simulink model "PBVS"  (R2020b)
settings: Solver=VariableStepAuto  StartTime=0.0  StopTime=7  RelTol=1e-3
values from neighbouring files (symbols this model uses):
  beta = 0.01    [init_PBVS.m]
  dT = 1/frequency    (= 0.005)    [init.m]    (also in init_PBVS.m = 0.002)
  DT = 1/20    (= 0.05)    [init_PBVS.m]
  f = 0.5    [init.m]    (also in init_PBVS.m = 0.1; robotIK.m = zeros(3,1))
  init_pose = [C ; ang']    [init.m]    (also in init_PBVS.m = [position(1:3); orientation'])
  Kd = 0.1*eye(6)    [init_PBVS.m]
  Kp = 1*eye(6)    [init.m]    (also in init_PBVS.m = diag([4 4 4 1.5 1.5 1.5]))
  N = 10    [init_PBVS.m]    (also in robotIK.m = size(jointLim, 1); workspace.m = 50)
  O = [0; 0; 0]    [init.m]    (also in init_PBVS.m)
  p = [0.25; 0; 0.25]    [init_PBVS.m]
  P0 = eye(6)*0.5    [init_PBVS.m]
  plane_x = 0.1    [init_PBVS.m]
  plane_y = 0.08    [init_PBVS.m]
  q = [0. 0. 0. -pi/2 0. pi/2 0. 0 0.]    [init_PBVS.m]    (also in robotIK.m = real(qToCheck))
  Q = zeros(6)    [init_PBVS.m]
  ref = [-0.2; 0; 0; pi/2; 0 ; pi/2]    [init.m]    (also in init_PBVS.m = [0; 0; 0.15; 0;  0; -pi])
libraries: simulink x2, robotmaniplib x2, cstblocks x1
settings Model: Creator=Acer  LastModifiedBy=antonio

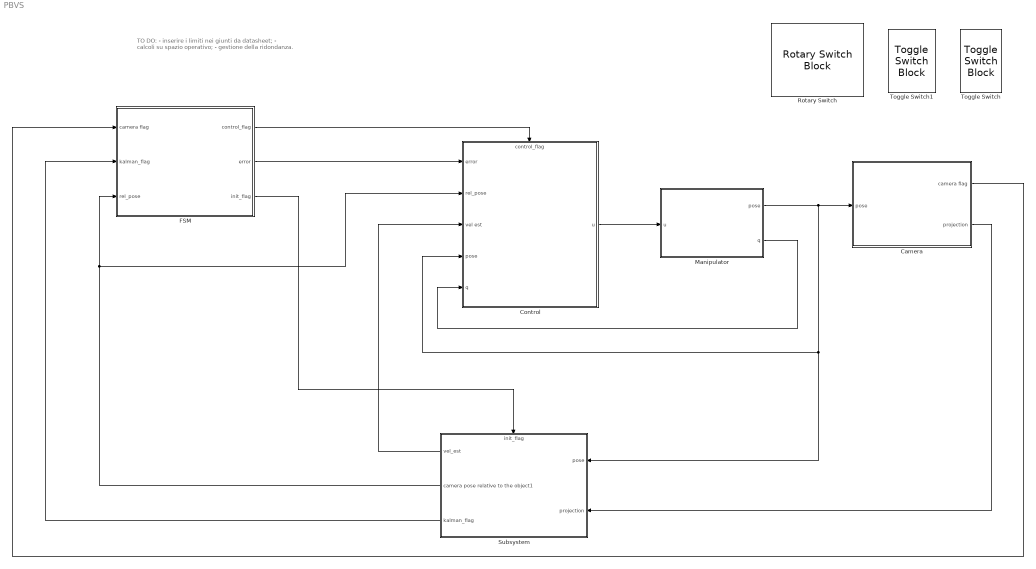
== system PBVS ==
  note: TO DO:
      | - inserire i limiti nei giunti da datasheet;
      | - calcoli su spazio operativo;
      | - gestione della ridondanza.
  Camera : Subsystem
  Control : Subsystem
      settings: PortSchema="{\"entries\":[{\"content\":{\"sides\":[{\"content\":{\"connectorIds\":[\"In1\",\"In2\",\"In3\",\"In4\",\"In5\"]},\"type\":\"ConnectorPlacement.EquallySpacedRectSide\",\"uuid\":\"af17fae2-36f6-4efd-b4ba-fb8d1f73429e\"},{\"content\":{\"connectorIds\":[\"Out1\"],\"side\":\"RIGHT\"},\"type\":\"ConnectorPlacement.EquallySpacedRectSide\",\"uuid\":\"2b8fdab6-bdef-4319-b746-176742d42689\"},{\"content\":{\"connectorIds\":[\"In6\"],\"side\":\"TOP\"},\"type\":\"ConnectorPlacement.EquallySpacedRectSide\",\"uuid\":\"e47b4a6a-66e6-45a0-98f9-e5ee84c20568\"},{\"content\":{\"connectorIds\":[],\"side\":\"HIDDEN\"},\"type\":\"ConnectorPlacement.EquallySpacedRectSide\",\"uuid\":\"9d3dc715-f15e-4844-9864-7097570c16fc\"}]},\"type\":\"ConnectorPlacement.EquallySpacedConnector\",\"uuid\":\"752007b5-316d-48d1-9942-1c7a203faf23\"}],\"packageUris\":[\"http://schema.mathworks.com/mf0/Connector/R2020b\"],\"version\":\"1.0\"}"
  FSM : Subsystem
  Manipulator : Subsystem
  Rotary Switch : RotarySwitchBlock  LabelPosition=Bottom
      settings: Values={{'Off', 'Low', 'Medium', 'High'}, [0 -0.03 -0.06 -0.1]}
  Subsystem : Subsystem
      settings: PortSchema="{\"entries\":[{\"content\":{\"sides\":[{\"content\":{\"connectorIds\":[\"In1\",\"In2\"]},\"type\":\"ConnectorPlacement.EquallySpacedRectSide\",\"uuid\":\"a08c32dc-abe6-4f2b-ae77-c4d2f876d1ca\"},{\"content\":{\"connectorIds\":[\"Out1\",\"Out2\",\"Out3\"],\"side\":\"RIGHT\"},\"type\":\"ConnectorPlacement.EquallySpacedRectSide\",\"uuid\":\"a9594212-1ad7-4004-b7e9-4ae8430051bc\"},{\"content\":{\"connectorIds\":[\"In3\"],\"side\":\"TOP\"},\"type\":\"ConnectorPlacement.EquallySpacedRectSide\",\"uuid\":\"c64d48d0-945a-48a3-9b1a-7425a2bac4f1\"},{\"content\":{\"connectorIds\":[],\"side\":\"HIDDEN\"},\"type\":\"ConnectorPlacement.EquallySpacedRectSide\",\"uuid\":\"141999d7-d8a1-4566-a0df-60055f832239\"}]},\"type\":\"ConnectorPlacement.EquallySpacedConnector\",\"uuid\":\"574f16a2-9616-413e-b861-7d1dd0d71272\"}],\"packageUris\":[\"http://schema.mathworks.com/mf0/Connector/R2020b\"],\"version\":\"1.0\"}"
  Toggle Switch : ToggleSwitchBlock  LabelPosition=Bottom
      settings: Values={{'Off', 'On'}, [0 1]}
  Toggle Switch1 : ToggleSwitchBlock  LabelPosition=Bottom
      settings: Values={{'Off', 'On'}, [0 1]}
  wires:
  Camera/2(projection) -> Subsystem/2(projection)
  Control/1(u) -> Manipulator/1(u)
  Manipulator/1(pose) -> Subsystem/1(pose), Control/4(pose), Camera/1(pose)
  Manipulator/2(q) -> Control/5(q)
  Subsystem/2(camera pose relative to the object1) -> FSM/3(rel_pose), Control/2(rel_pose)
  Subsystem/1(vel_est) -> Control/3(vel est)
  FSM/2(error) -> Control/1(error)
  Subsystem/3(kalman_flag) -> FSM/2(kalman_flag)
  FSM/1(control_flag) -> Control/6(control_flag)
  FSM/3(init_flag) -> Subsystem/3(init_flag)
  Camera/1(camera flag) -> FSM/1(camera flag)

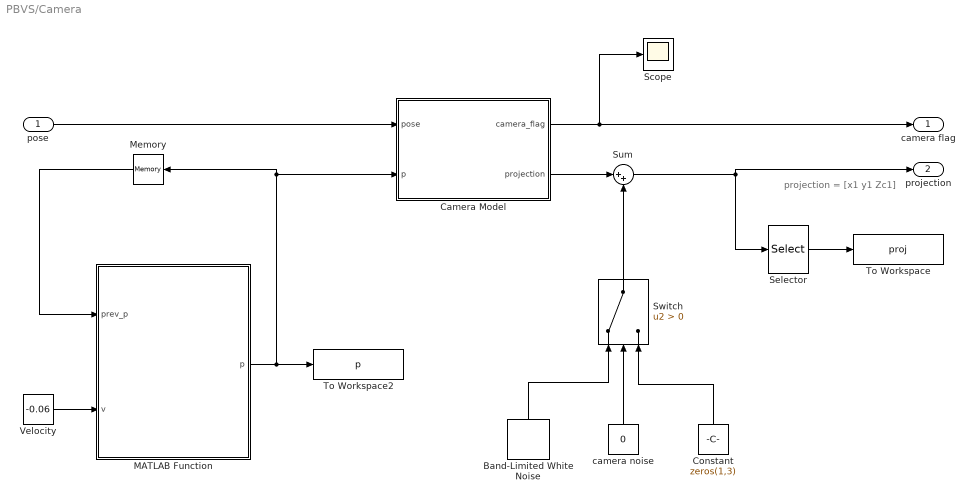
== system PBVS/Camera ==
  note: projection = [x1 y1 Zc1]
  pose : Inport
  Band-Limited White Noise : simulink/Sources/Band-Limited White Noise  Cov=[0.000001 0.000001 0.000001]  Ts=0.01  seed=[23341 10 14]
  Camera Model : MATLAB Function  TreatAsAtomicUnit=on
  Constant : Constant  Value=zeros(1,3)
  MATLAB Function : MATLAB Function  TreatAsAtomicUnit=on  SystemSampleTime=dT
  Memory : Memory  InitialCondition=[p]
  Scope : Scope
  Selector : Selector  InputPortWidth=3  IndexOptions=Index vector (dialog)  Indices=[1 2]  OutputSizes=1
  Sum : Sum  Inputs=|++
  Switch : Switch  Criteria=u2 > Threshold
  To Workspace : ToWorkspace  VariableName=proj  SampleTime=0.1
  To Workspace2 : ToWorkspace  VariableName=p  SampleTime=0.1
  Velocity : Constant  Value=-0.06  SampleTime=dT
  camera noise : Constant  Value=0
  camera flag : Outport
  projection : Outport  Port=2
  wires:
  pose/1 -> Camera Model/1(pose)
  Selector/1 -> To Workspace/1
  Camera Model/2(projection) -> Sum/1
  Sum/1 -> projection/1, Selector/1
  Switch/1 -> Sum/2
  camera noise/1 -> Switch/2
  Band-Limited White Noise/1 -> Switch/1
  Constant/1 -> Switch/3
  MATLAB Function/1(p) -> To Workspace2/1, Memory/1, Camera Model/2(p)
  Memory/1 -> MATLAB Function/1(prev_p)
  Velocity/1 -> MATLAB Function/2(v)
  Camera Model/1(camera_flag) -> Scope/1, camera flag/1

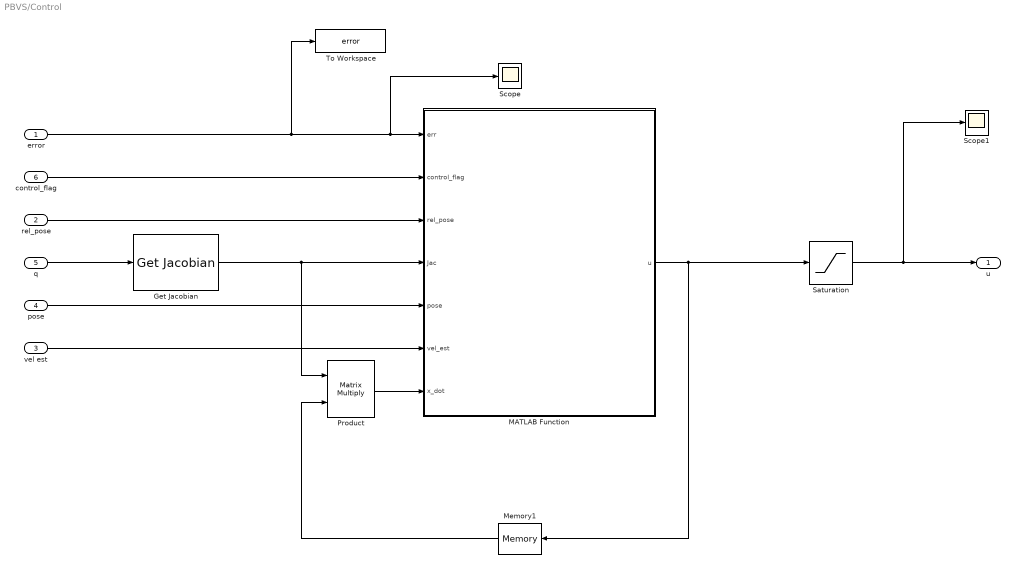
== system PBVS/Control ==
  error : Inport
  rel_pose : Inport  Port=2
  vel est : Inport  Port=3
  pose : Inport  Port=4
  q : Inport  Port=5
  control_flag : Inport  Port=6
  Get Jacobian : robotmaniplib/Get Jacobian  RigidBodyTree=robot  EndEffector=panda_hand  SimulateUsing=Interpreted execution
      settings: SourceProductBaseCode=RO
  MATLAB Function : MATLAB Function  TreatAsAtomicUnit=on  SystemSampleTime=dT
  Memory1 : Memory  InitialCondition=zeros(9,1)
  Product : Product  Multiplication=Matrix(*)
  Saturation : Saturate  UpperLimit=2.5  LowerLimit=-2.5
  Scope : Scope
  Scope1 : Scope
  To Workspace : ToWorkspace  VariableName=error  SampleTime=0.1
  u : Outport
  wires:
  error/1 -> To Workspace/1, Scope/1, MATLAB Function/1(err)
  rel_pose/1 -> MATLAB Function/3(rel_pose)
  MATLAB Function/1(u) -> Memory1/1, Saturation/1
  q/1 -> Get Jacobian/1
  Get Jacobian/1 -> Product/1, MATLAB Function/4(Jac)
  Saturation/1 -> Scope1/1, u/1
  pose/1 -> MATLAB Function/5(pose)
  Product/1 -> MATLAB Function/7(x_dot)
  Memory1/1 -> Product/2
  vel est/1 -> MATLAB Function/6(vel_est)
  control_flag/1 -> MATLAB Function/2(control_flag)

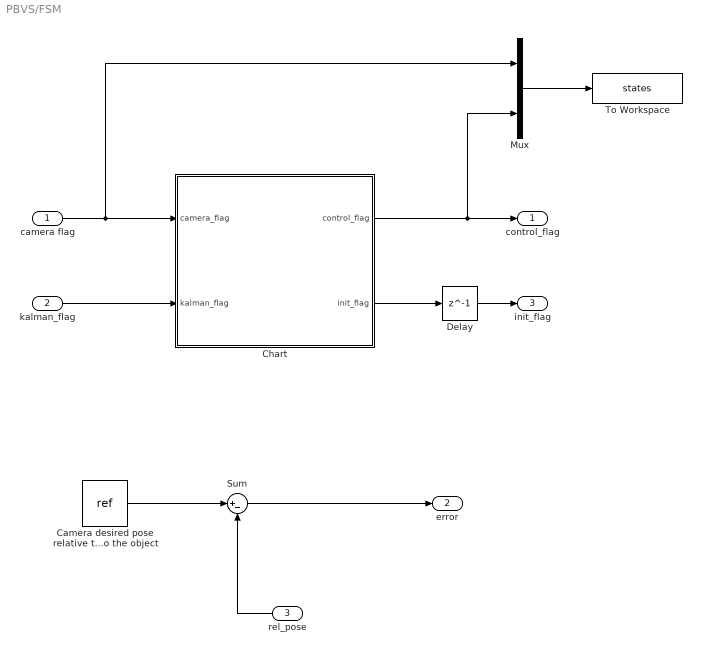
== system PBVS/FSM ==
  camera flag : Inport
  kalman_flag : Inport  Port=2
  rel_pose : Inport  Port=3
  Camera desired pose relative to the object : Constant  Value=ref  SampleTime=-1
  Chart : Stateflow chart  TreatAsAtomicUnit=on
  Delay : Delay  DelayLength=1
  Mux : Mux  Inputs=2
  Sum : Sum  Inputs=|+-
  To Workspace : ToWorkspace  VariableName=states  SampleTime=0.1
  control_flag : Outport
  error : Outport  Port=2
  init_flag : Outport  Port=3
  wires:
  Sum/1 -> error/1
  Camera desired pose relative to the object/1 -> Sum/1
  rel_pose/1 -> Sum/2
  kalman_flag/1 -> Chart/2(kalman_flag)
  Chart/1(control_flag) -> Mux/2, control_flag/1
  camera flag/1 -> Chart/1(camera_flag), Mux/1
  Chart/2(init_flag) -> Delay/1
  Delay/1 -> init_flag/1
  Mux/1 -> To Workspace/1

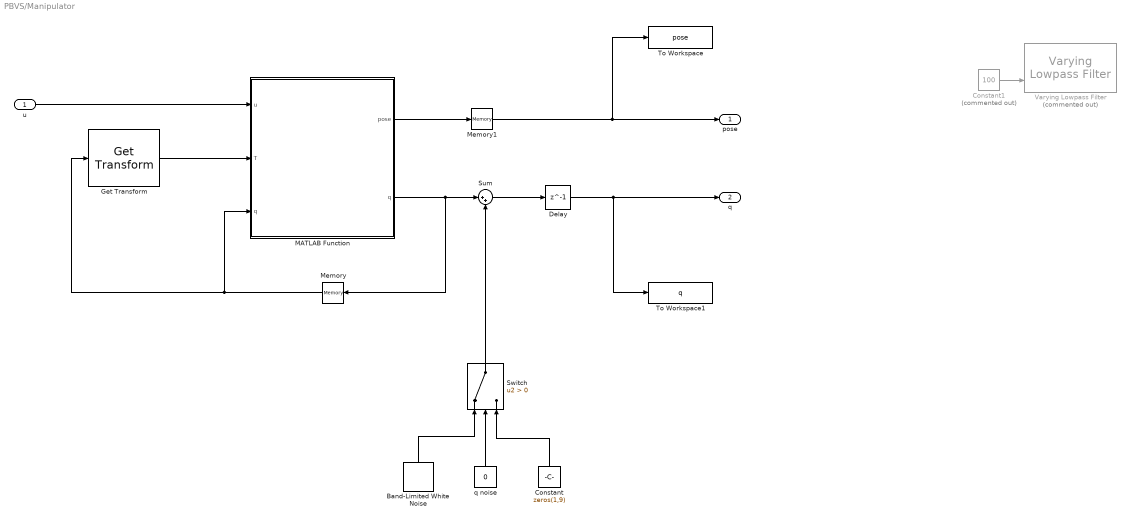
== system PBVS/Manipulator ==
  u : Inport
  Band-Limited White Noise : simulink/Sources/Band-Limited White Noise  Cov=[0.000001 0.000001 0.000001 0.000001 0.000001 0.000001 0.000001 0.0 0.0]  Ts=0.01  seed=[3341 17 144 12 1 94 2456 78 91]
  Constant : Constant  Value=zeros(1,9)
  Constant1 : Constant  Commented=on  Value=100
  Delay : Delay  DelayLength=1
  Get Transform : robotmaniplib/Get Transform  RigidBodyTree=robot  SourceBody=panda_link0  TargetBody=panda_hand  SimulateUsing=Interpreted execution
  MATLAB Function : MATLAB Function  TreatAsAtomicUnit=on  SystemSampleTime=dT
  Memory : Memory  InitialCondition=q
  Memory1 : Memory  InitialCondition=init_pose
  Sum : Sum  Inputs=|++
  Switch : Switch  Criteria=u2 > Threshold
  To Workspace : ToWorkspace  VariableName=pose  SampleTime=0.1
  To Workspace1 : ToWorkspace  VariableName=q  SampleTime=0.1
  Varying Lowpass Filter : cstblocks/Linear Parameter Varying/Varying Lowpass Filter  Commented=on  N=1
  q noise : Constant  Value=0
  pose : Outport
  q : Outport  Port=2
  wires:
  Memory/1 -> MATLAB Function/3("q "), Get Transform/1
  Get Transform/1 -> MATLAB Function/2(T)
  MATLAB Function/1(pose) -> Memory1/1
  Memory1/1 -> pose/1, To Workspace/1
  u/1 -> MATLAB Function/1(u)
  Constant/1 -> Switch/3
  Band-Limited White Noise/1 -> Switch/1
  Switch/1 -> Sum/2
  q noise/1 -> Switch/2
  MATLAB Function/2(q) -> Memory/1, Sum/1
  Sum/1 -> Delay/1
  Delay/1 -> q/1, To Workspace1/1
  Constant1/1 -> Varying Lowpass Filter/2

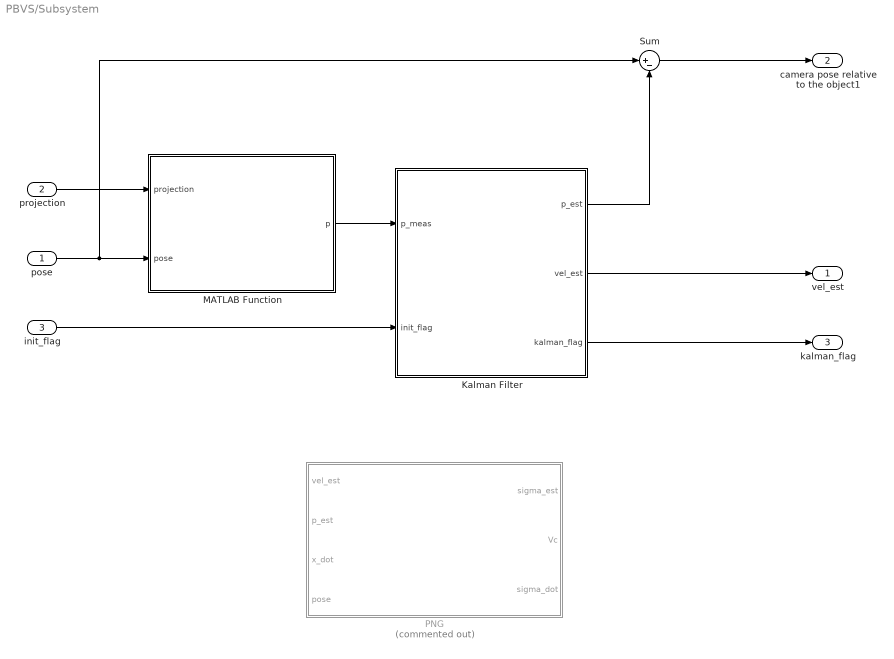
== system PBVS/Subsystem ==
  pose : Inport
  projection : Inport  Port=2
  init_flag : Inport  Port=3
  Kalman Filter : Subsystem
  MATLAB Function : MATLAB Function  TreatAsAtomicUnit=on
  PNG : Subsystem  Commented=on
  Sum : Sum  Inputs=|+-
  vel_est : Outport
  camera pose relative to the object1 : Outport  Port=2
  kalman_flag : Outport  Port=3
  wires:
  projection/1 -> MATLAB Function/1(projection)
  MATLAB Function/1(p) -> Kalman Filter/1(p_meas)
  Kalman Filter/2(vel_est) -> vel_est/1
  pose/1 -> Sum/1, MATLAB Function/2(pose)
  Sum/1 -> camera pose relative to the object1/1
  Kalman Filter/1(p_est) -> Sum/2
  Kalman Filter/3(kalman_flag) -> kalman_flag/1
  init_flag/1 -> Kalman Filter/2(init_flag)

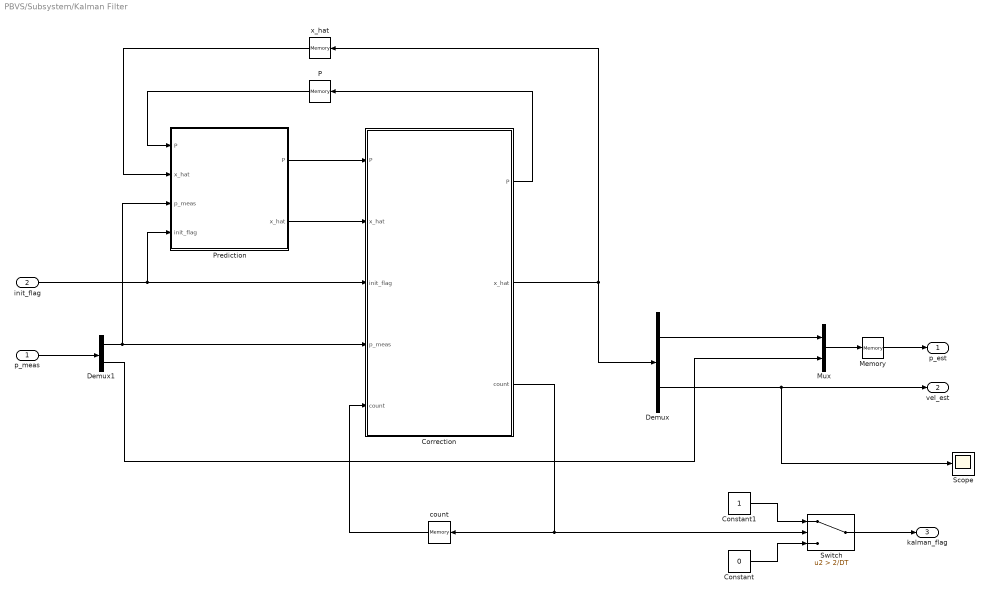
== system PBVS/Subsystem/Kalman Filter ==
  p_meas : Inport
  init_flag : Inport  Port=2
  Constant : Constant  Value=0
  Constant1 : Constant
  Correction : MATLAB Function  TreatAsAtomicUnit=on  SystemSampleTime=DT
  Demux : Demux  Outputs=2
  Demux1 : Demux  Outputs=2
  Memory : Memory  InitialCondition=zeros(6,1)
  Mux : Mux  Inputs=2
  P : Memory  InitialCondition=P0
  Prediction : MATLAB Function  TreatAsAtomicUnit=on  SystemSampleTime=DT
  Scope : Scope
  Switch : Switch  Criteria=u2 > Threshold  Threshold=2/DT
  count : Memory
  x_hat : Memory  InitialCondition=[p; zeros(3,1)]
  p_est : Outport
  vel_est : Outport  Port=2
  kalman_flag : Outport  Port=3
  wires:
  Demux/2 -> Scope/1, vel_est/1
  x_hat/1 -> Prediction/2("x_hat ")
  P/1 -> Prediction/1("P ")
  Correction/2(x_hat) -> x_hat/1, Demux/1
  Correction/1(P) -> P/1
  Prediction/1(P) -> Correction/1("P ")
  Prediction/2(x_hat) -> Correction/2("x_hat ")
  p_meas/1 -> Demux1/1
  Mux/1 -> Memory/1
  Demux/1 -> Mux/1
  Demux1/1 -> Prediction/3(p_meas), Correction/4(p_meas)
  Demux1/2 -> Mux/2
  Memory/1 -> p_est/1
  Correction/3(count) -> count/1, Switch/2
  count/1 -> Correction/5("count ")
  Constant/1 -> Switch/3
  Constant1/1 -> Switch/1
  Switch/1 -> kalman_flag/1
  init_flag/1 -> Prediction/4(init_flag), Correction/3(init_flag)

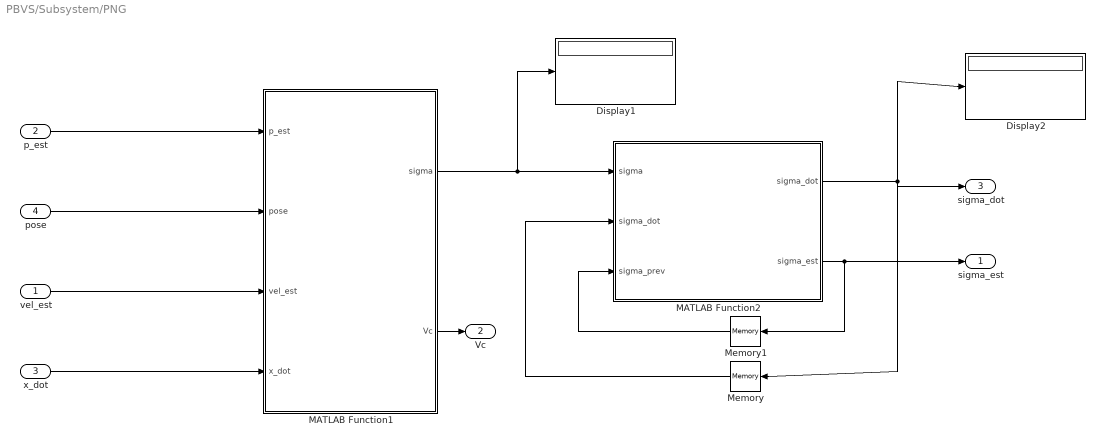
== system PBVS/Subsystem/PNG ==
  vel_est : Inport
  p_est : Inport  Port=2
  x_dot : Inport  Port=3
  pose : Inport  Port=4
  Display1 : Display
  Display2 : Display
  MATLAB Function1 : MATLAB Function  TreatAsAtomicUnit=on
  MATLAB Function2 : MATLAB Function  TreatAsAtomicUnit=on  SystemSampleTime=DT
  Memory : Memory  InitialCondition=zeros(3,1)
  Memory1 : Memory  InitialCondition=zeros(3,1)
  sigma_est : Outport
  Vc : Outport  Port=2
  sigma_dot : Outport  Port=3
  wires:
  MATLAB Function1/2(Vc) -> Vc/1
  MATLAB Function2/2(sigma_est) -> sigma_est/1, Memory1/1
  MATLAB Function1/1(sigma) -> Display1/1, MATLAB Function2/1(sigma)
  pose/1 -> MATLAB Function1/2(pose)
  Memory/1 -> MATLAB Function2/2("sigma_dot ")
  MATLAB Function2/1(sigma_dot) -> sigma_dot/1, Display2/1, Memory/1
  Memory1/1 -> MATLAB Function2/3(sigma_prev)
  x_dot/1 -> MATLAB Function1/4(x_dot)
  p_est/1 -> MATLAB Function1/1(p_est)
  vel_est/1 -> MATLAB Function1/3(vel_est)

== stateflow chart PBVS/FSM/Chart ==
  state Stop
    entry:
    control_flag = 0;
    init_flag = 0;
  state ComputeSpeed
    entry:
    control_flag = 0;
    init_flag = 1;
  state GraspTheObject
    entry:
    control_flag = 1;
  (default) -> Stop
  ComputeSpeed -> Stop [order 2] : [camera_flag == 0]
  Stop -> ComputeSpeed : [camera_flag == 1]
  ComputeSpeed -> GraspTheObject [order 1] : [kalman_flag == 1]
  data: camera_flag input; kalman_flag input; control_flag output; init_flag output

== matlab function PBVS/Subsystem/PNG/MATLAB Function2 ==
  data: sigma input; sigma_dot output; sigma_dot input; sigma_prev input; sigma_est output; DT parameter; beta parameter
function [sigma_dot, sigma_est] = fading_filter(sigma, sigma_dot, sigma_prev, DT, beta)

G = 1 - beta^2;
H = (1 - beta)^2;
sigma_est = zeros(3,1);

sigma_est = sigma_prev + sigma_dot * DT + G * (sigma - (sigma_prev + sigma_dot*DT));
sigma_dot = sigma_dot + H/DT * (sigma - (sigma_prev + sigma_dot * DT))

== matlab function PBVS/Subsystem/Kalman Filter/Correction ==
  data: P input; P output; x_hat input; init_flag input; x_hat output; p_meas input; count input; R parameter; count output
function [P, x_hat, count] = correction(P, x_hat, init_flag,p_meas, count, R)

if init_flag == 1
C = [eye(3) zeros(3); zeros(3) zeros(3)];
z = [p_meas; zeros(3,1)];

K = P * C' * (C * P * C' + R)^-1;
x_hat = x_hat + K * (z - C * x_hat);
P = (eye(6) - K * C) * P;

count = count + 1;
end

== matlab function PBVS/Subsystem/Kalman Filter/Prediction ==
  data: P input; P output; x_hat input; p_meas input; x_hat output; Q parameter; DT parameter; init_flag input
function [P, x_hat] = prediction(P, x_hat, p_meas, Q, DT, init_flag)

if init_flag == 1
A = [eye(3) DT*eye(3); zeros(3) eye(3)];

x_hat = A * x_hat;
P = A * P * A' + Q;
end

== matlab function PBVS/Control/MATLAB Function ==
  data: err input; control_flag input; rel_pose input; Jac input; Kp parameter; u output; ref parameter; pose input; vel_est input; x_dot input; Kd parameter; dT parameter; N parameter
function u = fcn(err, control_flag, rel_pose, Jac, Kp, ref, pose, vel_est, x_dot, Kd, dT, N)

% rel_pose : relative pose between camera and object
% ref : desired relative pose between camera and object
% err : error between desired and actual pose of the camera relative to the object
u = zeros(9, 1);

if (control_flag == 1)

    ang = zeros(3, 1);
    J = zeros(6, 9);
    ang(1) = rel_pose(4) - ref(4);  % camera's orientation 
    ang(2) = rel_pose(5) - ref(5);
    ang(3) = rel_pose(6) - ref(6);

    %% Trasformation
    Rx = [1   0       0   ;
          0 cos(ang(1)) -sin(ang(1));
          0 sin(ang(1)) cos(ang(1))];

    Ry = [cos(ang(2)) 0 sin(ang(2)) ;
           0     1   0    ;
         -sin(ang(2)) 0 cos(ang(2))];

    Rz = [cos(ang(3)) -sin(ang(3)) 0;
          sin(ang(3))  cos(ang(3)) 0;
           0      0     1];

    Rd = Rz * Ry * Rx; % rotation matrix 

    J2 = [1     sin(ang(1))*tan(ang(2))    cos(ang(1))*tan(ang(2));
          0           cos(ang(1))                  -sin(ang(1));
          0     sin(ang(1))/cos(ang(2))    cos(ang(1))/cos(ang(2)) ];

    Ta = [0     -sin(pose(1))       cos(pose(1))*sin(pose(2));
          0      cos(pose(1))       sin(pose(1))*sin(pose(2));
          1          0                        cos(pose(2))];

    if (det(Ta)==0)
        Ta = eye(3);
    end

    %% Jacobian
    %J = eye(6);  % Jacobian J(q)
    J(1:3, :) = Jac(4:6, :);
    J(4:6, :) = Jac(1:3, :);
    %
    Ja = [eye(3) zeros(3); zeros(3) Rd'*Ta^-1] * J;
    %null_Ja = null(Ja);

    %% PBVS control Law
    % n = zeros(3,1);    % end effector acceleration in xy, xz, yz planes
    % n = N * cross(Vc, sigma_dot);
    % 
    % a_ee = zeros(3,1);
    % a_ee(1) = -n(1) * sin(sigma(1)) - n(2) * sin(sigma(2));
    % a_ee(2) = n(1) * cos(sigma(1)) - n(3) * sin(sigma(3));
    % a_ee(3) = n(2) * cos(sigma(2)) - n(3) * cos(sigma(3));
    % u_png = [a_ee * dT; zeros(3,1)]


    u_vel = [vel_est ; zeros(3,1)]; % control correction to take into account the object velocity
    
    u = pinv(Ja) * (Kp * err - Kd * x_dot + u_vel); %+ (eye(7) - pinv(Ja)*Ja) * q0';   %  x_dot = J(q) * q_dot
end

== matlab function PBVS/Camera/Camera Model ==
  data: camera_flag output; projection output; f parameter; O parameter; pose input; p input; plane_y parameter; plane_x parameter
function [camera_flag, projection]= proj(f, O, pose, p, plane_y, plane_x)
% function that computes the projection of the point in the image plane
% f : focal lenght
% O : world origin frame
% pose: pose of the camera
% p : point position

camera_flag = 1;
d = pose(1:3) - O;    % camera's position in world frame
ang = pose(4:6);      % camera's orientation               


%%
Rx = [1   0       0   ;
      0 cos(ang(1)) -sin(ang(1));
      0 sin(ang(1)) cos(ang(1))];

Ry = [cos(ang(2)) 0 sin(ang(2)) ;
       0     1   0    ;
     -sin(ang(2)) 0 cos(ang(2))];
 
Rz = [cos(ang(3)) -sin(ang(3)) 0;
      sin(ang(3))  cos(ang(3)) 0;
       0      0     1];


Rc = Rz * Ry * Rx;


Twc = [Rc            d;
      zeros(1,3)     1];

%%
P = diag([f,f,1]) * [eye(3), zeros(3,1)]; % camera projection matrix

p_cam = Twc^-1 * [p; 1];   % point position in camera frame

p_tilde = P * p_cam;

x_proj = p_tilde(1)/p_cam(3);
y_proj = p_tilde(2)/p_cam(3);
Zc = p_cam(3);


projection  = [x_proj; y_proj; Zc]; %; x_proj2; y_proj2; Zc2];
% x_proj1, y_proj1 : point projection in image plane
% Zc1 : point depth in camera frame

if abs(x_proj) > plane_x || abs(y_proj) > plane_y   % check object visibility
    camera_flag = 0;
end
end

== matlab function PBVS/Manipulator/MATLAB Function ==
  data: u input; T input; q input; pose output; dT parameter; O parameter; q output
function [pose, q] = fcn(u, T, q, dT, O)

position = zeros(4, 1);
orientation = zeros(3, 1);
coder.extrinsic('tform2eul');

%% 
q = q + u * dT;

%%

position = T^-1 * [O; 1];
orientation = tform2eul(T^-1);
pose = [position(1:3); orientation];

== matlab function PBVS/Camera/MATLAB Function ==
  data: prev_p input; p output; v input; dT parameter
function p = fcn(prev_p ,v, dT)

p = prev_p;

p = p + [0; v; 0] * dT;

== matlab function PBVS/Subsystem/MATLAB Function ==
  data: projection input; p output; pose input; O parameter; f parameter
function p  = fcn(projection, pose, O, f)
% function that computes the point position in camera frame from the point
% projection in the image plane 
% pose : pose of the camera 

x = projection(1); % x projection in the image plane
y = projection(2); % y projection in the image plane 
Zc = projection(3); % point depth in camera frame 

d = pose(1:3) - O;    % camera's position in world frame
ang = pose(4:6);      % camera's orientation 

%%
Rx = [1   0       0   ;
      0 cos(ang(1)) -sin(ang(1));
      0 sin(ang(1)) cos(ang(1))];

Ry = [cos(ang(2)) 0 sin(ang(2)) ;
       0     1   0    ;
     -sin(ang(2)) 0 cos(ang(2))];
 
Rz = [cos(ang(3)) -sin(ang(3)) 0;
      sin(ang(3))  cos(ang(3)) 0;
       0      0     1];


Rc = Rz * Ry * Rx;


Twc = [Rc            d;
      zeros(1,3)     1];

P = diag([f,f,1]) * [eye(3), zeros(3,1)]; % camera projection matrix


p_tilde = [x * Zc; y * Zc; Zc];
p_cam = P(:, 1:3)^-1 * p_tilde;

p_hom = Twc * [p_cam; 1];
p = [p_hom(1:3); 0; 0; 0];   % [p1(1) p1(2) p1(3)] : point position in camera frame 
                               % [p1(4) p1(5) p1(6)] : point orientation in world frame 


% p1 = Twc * pinv(P) * [x1*Zc1; y1*Zc1; Zc1];
% p2 = Twc * pinv(P) * [x2*Zc2; y2*Zc2; Zc2];

== matlab function PBVS/Subsystem/PNG/MATLAB Function1 ==
  data: p_est input; pose input; vel_est input; x_dot input; sigma output; Vc output
function [sigma, Vc] = fcn(p_est, pose, vel_est, x_dot)

Ptm = zeros(3,1);
% Ptm(1) = p_est(1) - pose(1);
% Ptm(2) = p_est(2) - pose(2);
% Ptm(3) = p_est(3) - pose(3);
Ptm = p_est(1:3) - pose(1:3);
sigma = zeros(3,1);
sigma(1) = atan2(Ptm(2),Ptm(1));
sigma(2) = atan2(Ptm(3),Ptm(1));
sigma(3) = atan2(Ptm(3),Ptm(2));

Vtm = vel_est - x_dot(1:3); 

Vc = zeros(3,1);
Vc(1)= -(Ptm(1) * Vtm(1) + Ptm(2) * Vtm(2)) / (sqrt(Ptm(1)^2 + Ptm(2)^2)); % xy
Vc(2)= -(Ptm(1) * Vtm(1) + Ptm(3) * Vtm(3)) / (sqrt(Ptm(1)^2 + Ptm(3)^2)); % xz
Vc(3)= -(Ptm(2) * Vtm(2) + Ptm(3) * Vtm(3)) / (sqrt(Ptm(2)^2 + Ptm(3)^2)); % yz
